simulink subsystem "rss_MotoStallDiaSens"  (R2023a)
settings: Solver=VariableStepAuto  StartTime=0.0  StopTime=10.0  RelTol=1e-3
undefined symbols (not defined in the file): Cdbl_nElecAgSpdMaxVal, ENM_TYPE_FALT, Gs16_nMotoStallMinRefElecSpd_C, Gu16_ctMotoStallConfCnt_C, Gu16_ctMotoStallRcvyCnt_C
libraries: lib_debounce x1, lib_fault_definiteness x1
settings Model: Creator=xiaoqiang.yuan  LastModifiedBy=xiaoqiang.yuan

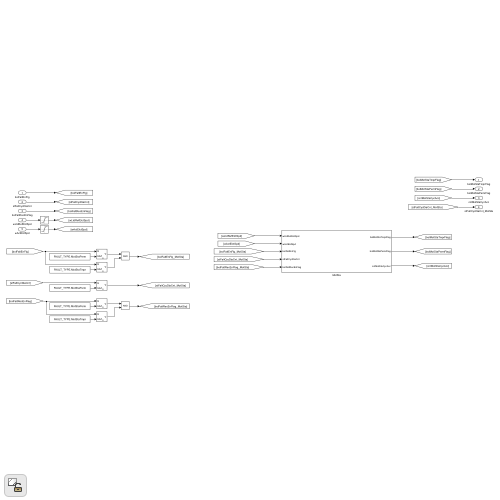
[thumbnail: Simulink's stored preview of the top-level diagram]
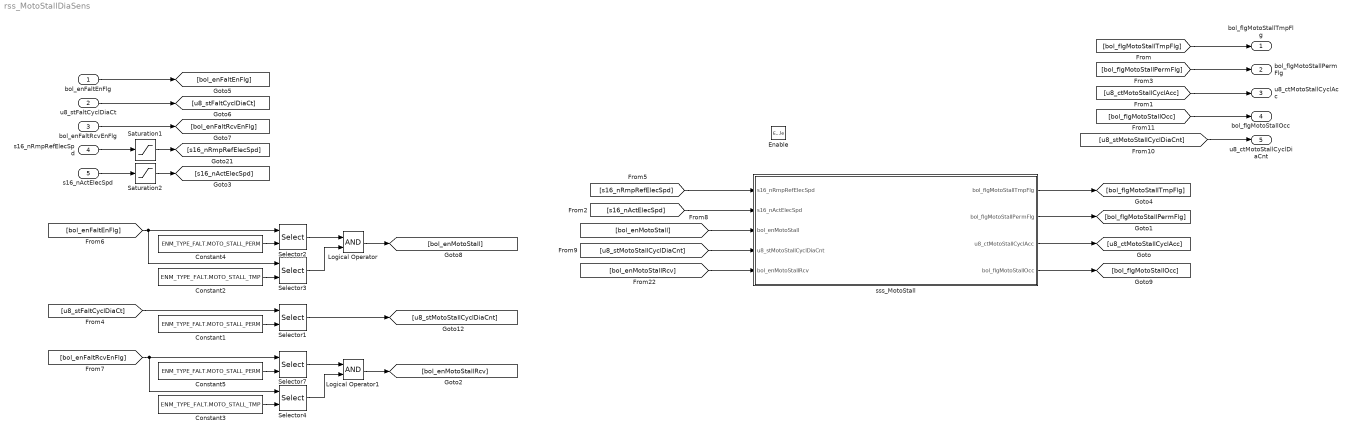
== system rss_MotoStallDiaSens ==
  bol_enFaltEnFlg : Inport  OutDataTypeStr=boolean
  u8_stFaltCyclDiaCt : Inport  Port=2  OutDataTypeStr=uint8
  bol_enFaltRcvEnFlg : Inport  Port=3  OutDataTypeStr=boolean
  s16_nRmpRefElecSpd : Inport  Port=4  OutDataTypeStr=dt_Standardize_s16p15b0
  s16_nActElecSpd : Inport  Port=5  OutDataTypeStr=dt_Standardize_s16p15b0
  Enable : EnablePort
  Constant1 : Constant  Value=ENM_TYPE_FALT.MOTO_STALL_PERM
  Constant2 : Constant  Value=ENM_TYPE_FALT.MOTO_STALL_TMP
  Constant3 : Constant  Value=ENM_TYPE_FALT.MOTO_STALL_TMP
  Constant4 : Constant  Value=ENM_TYPE_FALT.MOTO_STALL_PERM
  Constant5 : Constant  Value=ENM_TYPE_FALT.MOTO_STALL_PERM
  Logical Operator : Logic  AllPortsSameDT=off  OutDataTypeStr=boolean
  Logical Operator1 : Logic  AllPortsSameDT=off  OutDataTypeStr=boolean
  Saturation1 : Saturate  UpperLimit=Cdbl_nElecAgSpdMaxVal  LowerLimit=-Cdbl_nElecAgSpdMaxVal
  Saturation2 : Saturate  UpperLimit=Cdbl_nElecAgSpdMaxVal  LowerLimit=-Cdbl_nElecAgSpdMaxVal
  Selector{1..4,7} (5 alike) : Selector  IndexMode=Zero-based  InputPortWidth=Cdbl_numFaltDiaNum  IndexOptions=Index vector (port)  Indices=[1 3]  OutputSizes=1
  sss_MotoStall : Subsystem
  bol_flgMotoStallTmpFlg : Outport  OutDataTypeStr=boolean
  bol_flgMotoStallPermFlg : Outport  Port=2  OutDataTypeStr=boolean
  u8_ctMotoStallCyclAcc : Outport  Port=3  OutDataTypeStr=uint8
  bol_flgMotoStallOcc : Outport  Port=4  OutDataTypeStr=boolean
  u8_ctMotoStallCyclDiaCnt : Outport  Port=5  OutDataTypeStr=uint8
  wires:
  [bol_flgMotoStallTmpFlg] -> bol_flgMotoStallTmpFlg/1
  [u8_ctMotoStallCyclAcc] -> u8_ctMotoStallCyclAcc/1
  u8_stFaltCyclDiaCt/1 -> [u8_stFaltCyclDiaCt]
  [bol_enFaltRcvEnFlg] -> Selector7/1, Selector4/1
  s16_nActElecSpd/1 -> Saturation2/1
  s16_nRmpRefElecSpd/1 -> Saturation1/1
  [u8_stMotoStallCyclDiaCnt] -> sss_MotoStall/4(u8_stMotoStallCyclDiaCnt)
  Constant4/1 -> Selector2/2
  Constant5/1 -> Selector7/2
  Selector1/1 -> [u8_stMotoStallCyclDiaCnt]
  sss_MotoStall/1(bol_flgMotoStallTmpFlg) -> [bol_flgMotoStallTmpFlg]
  Constant1/1 -> Selector1/2
  bol_enFaltEnFlg/1 -> [bol_enFaltEnFlg]
  [bol_enMotoStallRcv] -> sss_MotoStall/5(bol_enMotoStallRcv)
  [s16_nRmpRefElecSpd] -> sss_MotoStall/1(s16_nRmpRefElecSpd)
  [bol_enMotoStall] -> sss_MotoStall/3(bol_enMotoStall)
  [bol_enFaltEnFlg] -> Selector2/1, Selector3/1
  [u8_stFaltCyclDiaCt] -> Selector1/1
  bol_enFaltRcvEnFlg/1 -> [bol_enFaltRcvEnFlg]
  [s16_nActElecSpd] -> sss_MotoStall/2(s16_nActElecSpd)
  sss_MotoStall/3(u8_ctMotoStallCyclAcc) -> [u8_ctMotoStallCyclAcc]
  sss_MotoStall/2(bol_flgMotoStallPermFlg) -> [bol_flgMotoStallPermFlg]
  [bol_flgMotoStallPermFlg] -> bol_flgMotoStallPermFlg/1
  Constant2/1 -> Selector3/2
  Selector2/1 -> Logical Operator/1
  Selector3/1 -> Logical Operator/2
  Logical Operator/1 -> [bol_enMotoStall]
  Constant3/1 -> Selector4/2
  Selector7/1 -> Logical Operator1/1
  Selector4/1 -> Logical Operator1/2
  Logical Operator1/1 -> [bol_enMotoStallRcv]
  [u8_stMotoStallCyclDiaCnt] -> u8_ctMotoStallCyclDiaCnt/1
  Saturation1/1 -> [s16_nRmpRefElecSpd]
  Saturation2/1 -> [s16_nActElecSpd]
  sss_MotoStall/4(bol_flgMotoStallOcc) -> [bol_flgMotoStallOcc]
  [bol_flgMotoStallOcc] -> bol_flgMotoStallOcc/1

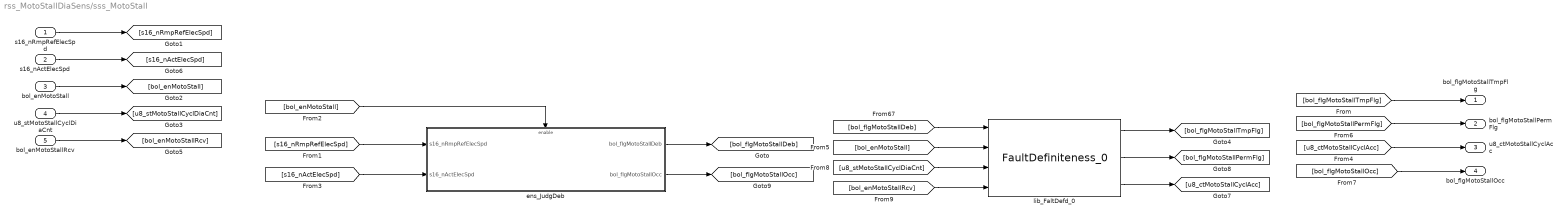
== system rss_MotoStallDiaSens/sss_MotoStall ==
  s16_nRmpRefElecSpd : Inport
  s16_nActElecSpd : Inport  Port=2
  bol_enMotoStall : Inport  Port=3
  u8_stMotoStallCyclDiaCnt : Inport  Port=4
  bol_enMotoStallRcv : Inport  Port=5
  ens_JudgDeb : Subsystem
  lib_FaltDefd_0 : lib_fault_definiteness/FaultDefiniteness_0  lb_FaltWaitRecvCnt=Gu16_ctMotoStallConfCnt_C
  bol_flgMotoStallTmpFlg : Outport
  bol_flgMotoStallPermFlg : Outport  Port=2
  u8_ctMotoStallCyclAcc : Outport  Port=3
  bol_flgMotoStallOcc : Outport  Port=4
  wires:
  [bol_flgMotoStallOcc] -> bol_flgMotoStallOcc/1
  ens_JudgDeb/2(bol_flgMotoStallOcc) -> [bol_flgMotoStallOcc]
  [s16_nActElecSpd] -> ens_JudgDeb/2(s16_nActElecSpd)
  lib_FaltDefd_0/2 -> [bol_flgMotoStallPermFlg]
  [bol_flgMotoStallPermFlg] -> bol_flgMotoStallPermFlg/1
  lib_FaltDefd_0/3 -> [u8_ctMotoStallCyclAcc]
  lib_FaltDefd_0/1 -> [bol_flgMotoStallTmpFlg]
  [u8_ctMotoStallCyclAcc] -> u8_ctMotoStallCyclAcc/1
  s16_nActElecSpd/1 -> [s16_nActElecSpd]
  [bol_enMotoStall] -> ens_JudgDeb/Enable
  [s16_nRmpRefElecSpd] -> ens_JudgDeb/1(s16_nRmpRefElecSpd)
  ens_JudgDeb/1(bol_flgMotoStallDeb) -> [bol_flgMotoStallDeb]
  bol_enMotoStallRcv/1 -> [bol_enMotoStallRcv]
  u8_stMotoStallCyclDiaCnt/1 -> [u8_stMotoStallCyclDiaCnt]
  bol_enMotoStall/1 -> [bol_enMotoStall]
  [bol_flgMotoStallTmpFlg] -> bol_flgMotoStallTmpFlg/1
  s16_nRmpRefElecSpd/1 -> [s16_nRmpRefElecSpd]
  [bol_enMotoStallRcv] -> lib_FaltDefd_0/4
  [u8_stMotoStallCyclDiaCnt] -> lib_FaltDefd_0/3
  [bol_enMotoStall] -> lib_FaltDefd_0/2
  [bol_flgMotoStallDeb] -> lib_FaltDefd_0/1

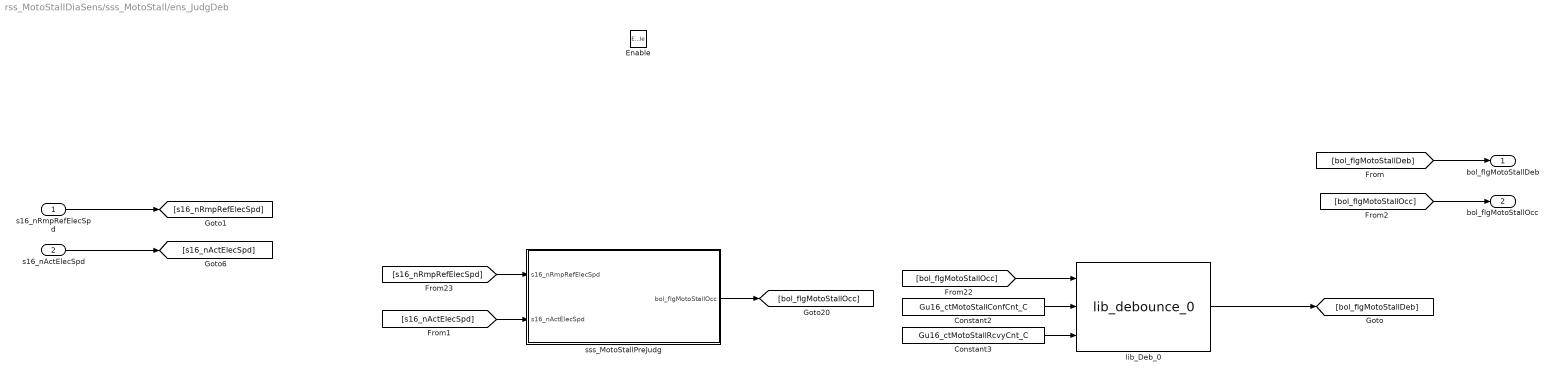
== system rss_MotoStallDiaSens/sss_MotoStall/ens_JudgDeb ==
  s16_nRmpRefElecSpd : Inport
  s16_nActElecSpd : Inport  Port=2
  Enable : EnablePort
  Constant2 : Constant  Value=Gu16_ctMotoStallConfCnt_C
  Constant3 : Constant  Value=Gu16_ctMotoStallRcvyCnt_C
  lib_Deb_0 : lib_debounce/lib_debounce_0
  sss_MotoStallPreJudg : Subsystem
  bol_flgMotoStallDeb : Outport
  bol_flgMotoStallOcc : Outport  Port=2
  wires:
  [bol_flgMotoStallOcc] -> bol_flgMotoStallOcc/1
  [s16_nActElecSpd] -> sss_MotoStallPreJudg/2(s16_nActElecSpd)
  s16_nActElecSpd/1 -> [s16_nActElecSpd]
  [s16_nRmpRefElecSpd] -> sss_MotoStallPreJudg/1(s16_nRmpRefElecSpd)
  s16_nRmpRefElecSpd/1 -> [s16_nRmpRefElecSpd]
  [bol_flgMotoStallDeb] -> bol_flgMotoStallDeb/1
  sss_MotoStallPreJudg/1(bol_flgMotoStallOcc) -> [bol_flgMotoStallOcc]
  Constant3/1 -> lib_Deb_0/3
  [bol_flgMotoStallOcc] -> lib_Deb_0/1
  lib_Deb_0/1 -> [bol_flgMotoStallDeb]
  Constant2/1 -> lib_Deb_0/2

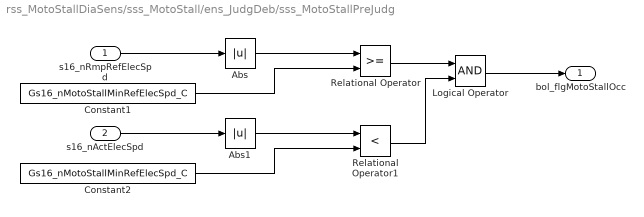
== system rss_MotoStallDiaSens/sss_MotoStall/ens_JudgDeb/sss_MotoStallPreJudg ==
  s16_nRmpRefElecSpd : Inport
  s16_nActElecSpd : Inport  Port=2
  Abs : Abs  SaturateOnIntegerOverflow=off
  Abs1 : Abs  SaturateOnIntegerOverflow=off
  Constant1 : Constant  Value=Gs16_nMotoStallMinRefElecSpd_C
  Constant2 : Constant  Value=Gs16_nMotoStallMinRefElecSpd_C
  Logical Operator : Logic  AllPortsSameDT=off  OutDataTypeStr=boolean
  Relational Operator : RelationalOperator  OutDataTypeStr=boolean  RndMeth=Simplest  InputSameDT=off
  Relational Operator1 : RelationalOperator  Operator=<  OutDataTypeStr=boolean  RndMeth=Simplest  InputSameDT=off
  bol_flgMotoStallOcc : Outport
  wires:
  Abs1/1 -> Relational Operator1/1
  Abs/1 -> Relational Operator/1
  Logical Operator/1 -> bol_flgMotoStallOcc/1
  Relational Operator1/1 -> Logical Operator/2
  Relational Operator/1 -> Logical Operator/1
  Constant2/1 -> Relational Operator1/2
  s16_nActElecSpd/1 -> Abs1/1
  Constant1/1 -> Relational Operator/2
  s16_nRmpRefElecSpd/1 -> Abs/1
